simulink model "Problem4_realize_filter"  (R2020b)
settings: Solver=VariableStepAuto  StartTime=0.0  StopTime=10  MaxStep=0.01  RelTol=1e-3
settings Model: Creator=vigne  LastModifiedBy=vigne

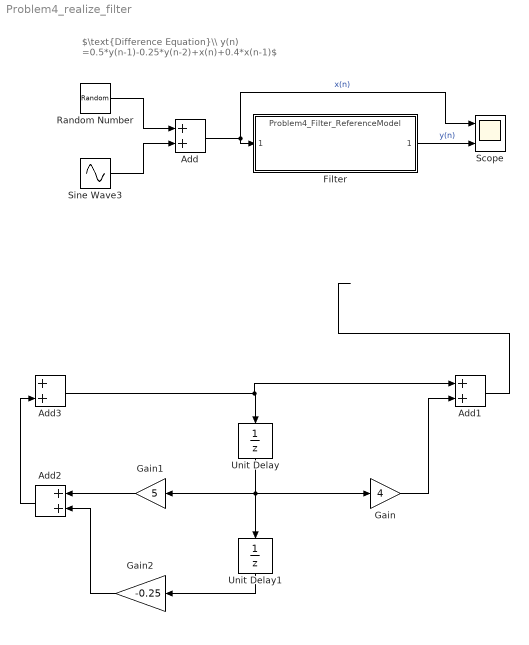
== system Problem4_realize_filter ==
  note: $\text{Difference Equation}\\ y(n) =0.5*y(n-1)-0.25*y(n-2)+x(n)+0.4*x(n-1)$
  Add{,1..3} (4 alike) : Sum
  Filter : ModelReference  ModelNameDialog=Problem4_Filter_ReferenceModel  SimulationMode=Normal  ModelReferenceVersion=1.10
  Gain : Gain  Gain=4
  Gain1 : Gain  Gain=5
  Gain2 : Gain  Gain=-0.25
  Random Number : RandomNumber  Variance=0.1  Seed=1  SampleTime=0.01
  Scope : Scope  NumInputPorts=2
  Sine Wave3 : Sin  Phase=2*pi*10000  SampleTime=0
  Unit Delay : UnitDelay  SampleTime=-1  HasFrameUpgradeWarning=on
  Unit Delay1 : UnitDelay  SampleTime=-1  HasFrameUpgradeWarning=on
  wires:
  Sine Wave3/1 -> Add/2
  Random Number/1 -> Add/1
  Add/1 -> Scope/1, Filter/1  "x(n)"
  Filter/1 -> Scope/2  "y(n)"
  Add2/1 -> Add3/2
  Add1/1 -> ?
  Add3/1 -> Add1/1, Unit Delay/1
  Unit Delay1/1 -> Gain2/1
  Gain1/1 -> Add2/1
  Gain/1 -> Add1/2
  Unit Delay/1 -> Gain/1, Unit Delay1/1, Gain1/1
  Gain2/1 -> Add2/2
  ? -> Add3/1
